simulink model "aula1403Sim"  (R2022a)
settings: Solver=VariableStepAuto  StartTime=0.0  StopTime=4  RelTol=1e-3
settings Model: Creator=a2270340  LastModifiedBy=a2270340

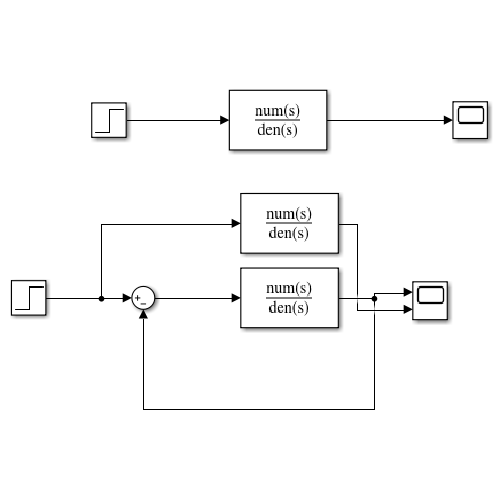
[thumbnail: Simulink's stored preview of the top-level diagram]
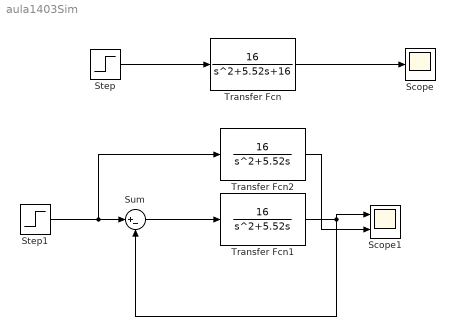
== system aula1403Sim ==
  Scope : Scope
  Scope1 : Scope  NumInputPorts=2
  Step : Step  Time=0  SampleTime=0
  Step1 : Step  Time=0  SampleTime=0
  Sum : Sum  Inputs=|+-
  Transfer Fcn : TransferFcn  Numerator=[16]  Denominator=[1 5.52 16]
  Transfer Fcn1 : TransferFcn  Numerator=[16]  Denominator=[1 5.52 0]
  Transfer Fcn2 : TransferFcn  Numerator=[16]  Denominator=[1 5.52 0]
  wires:
  Transfer Fcn/1 -> Scope/1
  Step/1 -> Transfer Fcn/1
  Sum/1 -> Transfer Fcn1/1
  Step1/1 -> Transfer Fcn2/1, Sum/1
  Transfer Fcn1/1 -> Sum/2, Scope1/1
  Transfer Fcn2/1 -> Scope1/2
